simulink model "hcs"  (Simulink 10.1)
settings: Solver=ode45  StartTime=0.0  StopTime=13  RelTol=1e-10  EnableMultiTasking=on
settings Model: Creator=liang  LastModifiedBy=bzhan
settings DataIOCC: LimitDataPoints=on  SignalLoggingSaveFormat=ModelDataLogs
settings OptimizationCC: ExpressionDepthLimit=2147483647
settings DebuggingCC: SolverPrmCheckMsg=warning  FcnCallInpInsideContextMsg=warning  StateNameClashWarn=warning
settings GRTTargetCC: CombineOutputUpdateFcns=on  GRTInterface=off

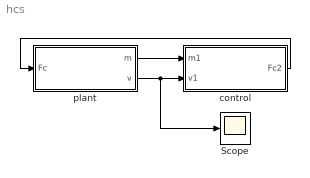
== system hcs ==
  Scope : Scope
  control : Subsystem
  plant : Subsystem
  wires:
  plant/1(m) -> control/1(m1)
  plant/2(v) -> Scope/1, control/2(v1)
  control/1(Fc2) -> plant/1(Fc)

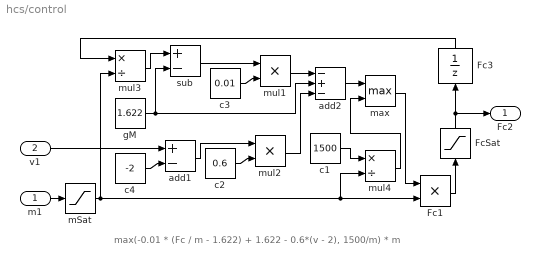
== system hcs/control ==
  note: max(-0.01 * (Fc / m - 1.622) + 1.622 - 0.6*(v - 2), 1500/m) * m
  m1 : Inport
  v1 : Inport  Port=2
  Fc1 : Product  Inputs=**  SampleTime=0.128
  Fc3 : UnitDelay  InitialCondition=2027.5  SampleTime=-1  HasFrameUpgradeWarning=on
  FcSat : Saturate  UpperLimit=5000  LowerLimit=1500  SampleTime=0.128
  add1 : Sum  Inputs=+-  SampleTime=0.128
  add2 : Sum  Inputs=-+-  SampleTime=0.128
  c1 : Constant  Value=1500
  c2 : Constant  Value=0.6
  c3 : Constant  Value=0.01
  c4 : Constant  Value=-2
  gM : Constant  Value=1.622
  mSat : Saturate  UpperLimit=3000  LowerLimit=1100  SampleTime=0.128
  max : MinMax  Function=max  Inputs=2  SampleTime=0.128
  mul1 : Product  Inputs=**  SampleTime=0.128
  mul2 : Product  Inputs=**  SampleTime=0.128
  mul3 : Product  Inputs=*/  SampleTime=0.128
  mul4 : Product  Inputs=*/  SampleTime=0.128
  sub : Sum  Inputs=+-  SampleTime=0.128
  Fc2 : Outport
  wires:
  m1/1 -> mSat/1
  mul3/1 -> sub/1
  gM/1 -> add2/2, sub/2
  sub/1 -> mul1/1
  c3/1 -> mul1/2
  c4/1 -> add1/2
  add1/1 -> mul2/1
  c2/1 -> mul2/2
  mul2/1 -> add2/3
  v1/1 -> add1/1
  add2/1 -> max/1
  Fc1/1 -> FcSat/1
  Fc3/1 -> mul3/1
  mul1/1 -> add2/1
  mSat/1 -> mul3/2, Fc1/2, mul4/2
  FcSat/1 -> Fc3/1, Fc2/1
  max/1 -> Fc1/1
  c1/1 -> mul4/1
  mul4/1 -> max/2

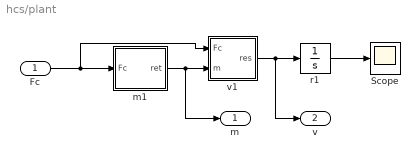
== system hcs/plant ==
  Fc : Inport
  Scope : Scope
  m1 : Subsystem
  r1 : Integrator  InitialCondition=30
  v1 : Subsystem
  m : Outport
  v : Outport  Port=2
  wires:
  m1/1(ret) -> v1/2(m), m/1
  v1/1(res) -> v/1, r1/1
  Fc/1 -> v1/1(Fc), m1/1(Fc)
  r1/1 -> Scope/1

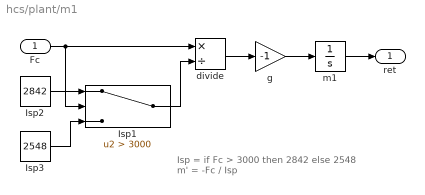
== system hcs/plant/m1 ==
  note: Isp = if Fc > 3000 then 2842 else 2548
      |
      | m' = -Fc / Isp
  Fc : Inport
  Isp1 : Switch  Criteria=u2 > Threshold  Threshold=3000  SampleTime=0
  Isp2 : Constant  Value=2842
  Isp3 : Constant  Value=2548
  divide : Product  Inputs=*/  SampleTime=0
  g : Gain  Gain=-1  SampleTime=0
  m1 : Integrator  InitialCondition=1250
  ret : Outport
  wires:
  Fc/1 -> divide/1, Isp1/2
  divide/1 -> g/1
  g/1 -> m1/1
  m1/1 -> ret/1
  Isp2/1 -> Isp1/1
  Isp3/1 -> Isp1/3
  Isp1/1 -> divide/2

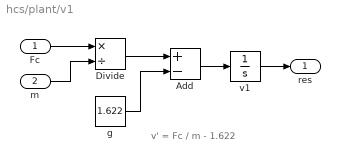
== system hcs/plant/v1 ==
  note: v' = Fc / m - 1.622
  Fc : Inport
  m : Inport  Port=2
  Add : Sum  Inputs=+-  SampleTime=0
  Divide : Product  Inputs=*/  SampleTime=0
  g : Constant  Value=1.622
  v1 : Integrator  InitialCondition=-2
  res : Outport
  wires:
  Fc/1 -> Divide/1
  m/1 -> Divide/2
  Divide/1 -> Add/1
  g/1 -> Add/2
  Add/1 -> v1/1
  v1/1 -> res/1
